simulink model "compare_preshaping"  (R2024b)
settings: Solver=VariableStepAuto  StartTime=0.0  StopTime=2  RelTol=1e-3
values from neighbouring files (symbols this model uses):
  a2 = shortened_step_value * 1/(1+K)    [simulate_preshaping.m]
  b2 = shortened_step_value    (= 15.923566879)    [simulate_preshaping.m]
  c2 = shortened_step_value * K/(1+K)    [simulate_preshaping.m]
  cruise_time = 1    [simulate_preshaping.m]
  deltaT = pi/(wn*sqrt(1-zeta^2))    [simulate_preshaping.m]
  initial_delay = 0.1    [simulate_preshaping.m]
  original_accel_time = 0.1    [simulate_preshaping.m]
  original_step_value = target_velocity / original_accel_time    (= 10)    [simulate_preshaping.m]
  shortened_step_time = 0.0628    [simulate_preshaping.m]
  tau = 0.1    [simulate_preshaping.m]
  wn = 100    [simulate_preshaping.m]
  zeta = 0.05    [simulate_preshaping.m]
settings Model: Creator=shohei  LastModifiedBy=shohei

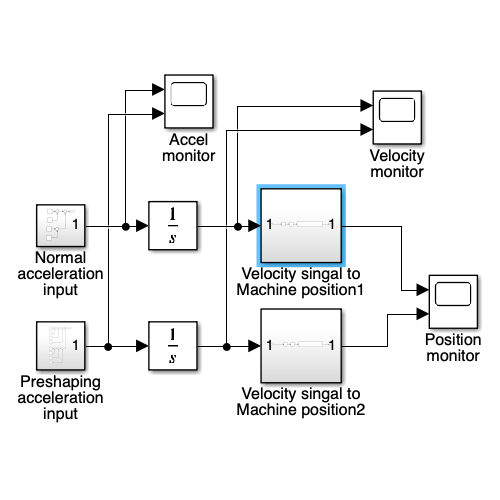
[thumbnail: Simulink's stored preview of the top-level diagram]
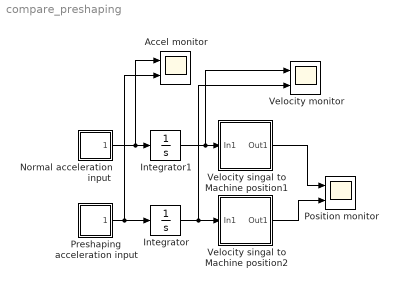
== system compare_preshaping ==
  Accel monitor : Scope  NumInputPorts=2
  Integrator : Integrator
  Integrator1 : Integrator
  Normal acceleration input : Subsystem
  Position monitor : Scope  NumInputPorts=2
  Preshaping acceleration input : Subsystem
  Velocity monitor : Scope  NumInputPorts=2
  Velocity singal to Machine position1 : Subsystem
  Velocity singal to Machine position2 : Subsystem
  wires:
  Preshaping acceleration input/1(Out1) -> Integrator/1, Accel monitor/2
  Normal acceleration input/1(Out1) -> Accel monitor/1, Integrator1/1
  Velocity singal to Machine position1/1(Out1) -> Position monitor/1
  Velocity singal to Machine position2/1(Out1) -> Position monitor/2
  Integrator/1 -> Velocity monitor/2, Velocity singal to Machine position2/1(In1)
  Integrator1/1 -> Velocity monitor/1, Velocity singal to Machine position1/1(In1)

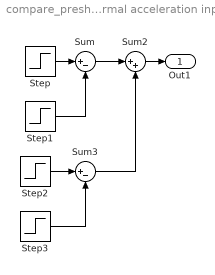
== system compare_preshaping/Normal acceleration input ==
  Step : Step  Time=initial_delay  After=original_step_value  SampleTime=0
  Step1 : Step  Time=initial_delay+original_accel_time  After=original_step_value  SampleTime=0
  Step2 : Step  Time=initial_delay+cruise_time  After=-original_step_value  SampleTime=0
  Step3 : Step  Time=initial_delay+cruise_time+original_accel_time  After=-original_step_value  SampleTime=0
  Sum : Sum  Inputs=|+-
  Sum2 : Sum  Inputs=|++
  Sum3 : Sum  Inputs=|+-
  Out1 : Outport
  wires:
  Sum2/1 -> Out1/1
  Sum3/1 -> Sum2/2
  Step2/1 -> Sum3/1
  Step/1 -> Sum/1
  Step3/1 -> Sum3/2
  Sum/1 -> Sum2/1
  Step1/1 -> Sum/2

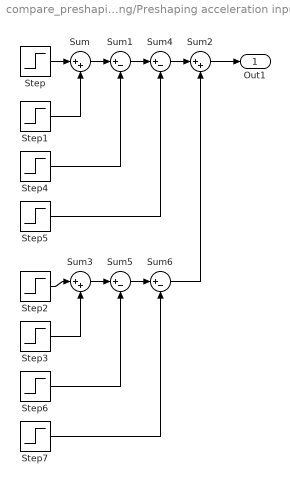
== system compare_preshaping/Preshaping acceleration input ==
  Step : Step  Time=initial_delay  After=a2  SampleTime=0
  Step1 : Step  Time=initial_delay+deltaT  After=b2-a2  SampleTime=0
  Step2 : Step  Time=initial_delay+cruise_time  After=-a2  SampleTime=0
  Step3 : Step  Time=initial_delay++cruise_time+deltaT  After=-(b2-a2)  SampleTime=0
  Step4 : Step  Time=initial_delay+shortened_step_time  After=a2  SampleTime=0
  Step5 : Step  Time=initial_delay+shortened_step_time+deltaT  After=c2  SampleTime=0
  Step6 : Step  Time=initial_delay++cruise_time+shortened_step_time  After=-a2  SampleTime=0
  Step7 : Step  Time=initial_delay++cruise_time+shortened_step_time+deltaT  After=-c2  SampleTime=0
  Sum : Sum  Inputs=|++
  Sum{1,4..6} (4 alike) : Sum  Inputs=|+-
  Sum2 : Sum  Inputs=|++
  Sum3 : Sum  Inputs=|++
  Out1 : Outport
  wires:
  Sum2/1 -> Out1/1
  Step4/1 -> Sum1/2
  Step7/1 -> Sum6/2
  Sum4/1 -> Sum2/1
  Sum1/1 -> Sum4/1
  Step3/1 -> Sum3/2
  Sum5/1 -> Sum6/1
  Step6/1 -> Sum5/2
  Step5/1 -> Sum4/2
  Step2/1 -> Sum3/1
  Sum3/1 -> Sum5/1
  Step/1 -> Sum/1
  Sum6/1 -> Sum2/2
  Sum/1 -> Sum1/1
  Step1/1 -> Sum/2

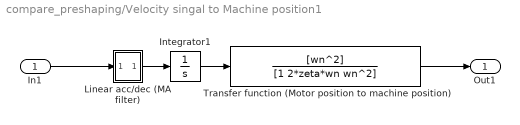
== system compare_preshaping/Velocity singal to Machine position1 ==
  In1 : Inport
  Integrator1 : Integrator
  Linear acc/dec (MA filter) : Subsystem
  Transfer function (Motor position to machine position) : TransferFcn  Numerator=[wn^2]  Denominator=[1 2*zeta*wn wn^2]
  Out1 : Outport
  wires:
  Transfer function (Motor position to machine position)/1 -> Out1/1
  Linear acc/dec (MA filter)/1(Out1) -> Integrator1/1
  Integrator1/1 -> Transfer function (Motor position to machine position)/1
  In1/1 -> Linear acc/dec (MA filter)/1(In1)

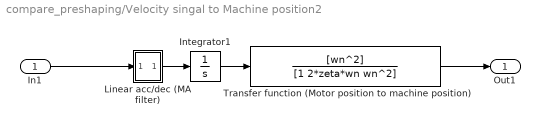
== system compare_preshaping/Velocity singal to Machine position2 ==
  In1 : Inport
  Integrator1 : Integrator
  Linear acc/dec (MA filter) : Subsystem
  Transfer function (Motor position to machine position) : TransferFcn  Numerator=[wn^2]  Denominator=[1 2*zeta*wn wn^2]
  Out1 : Outport
  wires:
  Transfer function (Motor position to machine position)/1 -> Out1/1
  Linear acc/dec (MA filter)/1(Out1) -> Integrator1/1
  Integrator1/1 -> Transfer function (Motor position to machine position)/1
  In1/1 -> Linear acc/dec (MA filter)/1(In1)

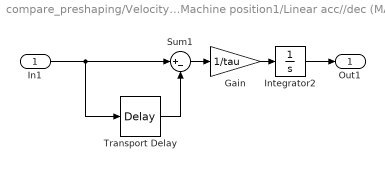
== system compare_preshaping/Velocity singal to Machine position1/Linear acc//dec (MA filter) ==
  In1 : Inport
  Gain : Gain  Gain=1/tau
  Integrator2 : Integrator
  Sum1 : Sum  Inputs=|+-
  Transport Delay : TransportDelay  DelayTime=tau
  Out1 : Outport
  wires:
  In1/1 -> Sum1/1, Transport Delay/1
  Integrator2/1 -> Out1/1
  Gain/1 -> Integrator2/1
  Sum1/1 -> Gain/1
  Transport Delay/1 -> Sum1/2

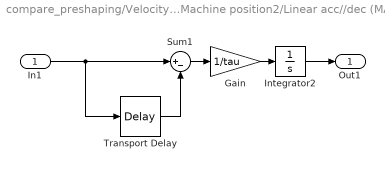
== system compare_preshaping/Velocity singal to Machine position2/Linear acc//dec (MA filter) ==
  In1 : Inport
  Gain : Gain  Gain=1/tau
  Integrator2 : Integrator
  Sum1 : Sum  Inputs=|+-
  Transport Delay : TransportDelay  DelayTime=tau
  Out1 : Outport
  wires:
  In1/1 -> Sum1/1, Transport Delay/1
  Integrator2/1 -> Out1/1
  Gain/1 -> Integrator2/1
  Sum1/1 -> Gain/1
  Transport Delay/1 -> Sum1/2
